simulink model "testSysObj"  (R2013b)
settings: Solver=FixedStepDiscrete  StartTime=0.0  StopTime=Inf  FixedStep=Ts  RelTol=1e-3
PreLoadFcn:
  | s1 = w32serial('COM8');
  | s2 = w32serial('COM40');
  | Ts = 1;
InitFcn:
  | if isequal(s1.CurrentState,'Opened')
  |     fclose(s1);
  | end
  | if isequal(s2.CurrentState,'Opened')
  |     fclose(s2);
  | end
  | 
  | fopen(s1);
  | fopen(s2);
StopFcn:
  | if isequal(s1.CurrentState,'Opened')
  |     fclose(s1);
  | end
  | if isequal(s2.CurrentState,'Opened')
  |     fclose(s2);
  | end
libraries: simulink x2, aerolibanimutils x1
settings Model: Creator=scastro  LastModifiedBy=scastro

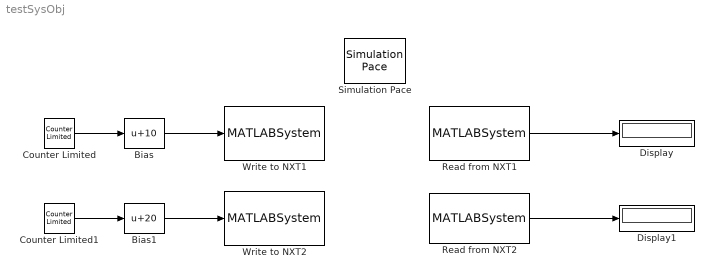
== system testSysObj ==
  Bias : Bias  Bias=10
  Bias1 : Bias  Bias=20
  Counter Limited : simulink/Sources/Counter Limited  uplimit=7  tsamp=Ts
  Counter Limited1 : simulink/Sources/Counter Limited  uplimit=7  tsamp=Ts
  Display : Display
  Display1 : Display
  Read from NXT1 : MATLABSystem  System=w32read  SimulateUsing=Interpreted execution  COMObj=s1  DataType=uint8  DataSize=1  DataLength=1  Mailbox=2
      mask Type: w32read
      mask Display:
      | disp('w32read');
      | port_label('output',1,'msg');
  Read from NXT2 : MATLABSystem  System=w32read  SimulateUsing=Interpreted execution  COMObj=s2  DataType=uint8  DataSize=1  DataLength=1  Mailbox=4
      mask Type: w32read
      mask Display:
      | disp('w32read');
      | port_label('output',1,'msg');
  Simulation Pace : aerolibanimutils/Simulation Pace  SimulationPace=1  SleepMode=MATLAB Thread  OutputPaceError=off  SampleTime=-1
      settings: AttributesFormatString=%<SimulationPace> sec/sec
  Write to NXT1 : MATLABSystem  System=w32write  SimulateUsing=Interpreted execution  COMObj=s1  DataType=uint8  DataSize=1  DataLength=1  Mailbox=1
      mask Type: w32write
      mask Display:
      | disp('w32write');
      | port_label('input',1,'data');
  Write to NXT2 : MATLABSystem  System=w32write  SimulateUsing=Interpreted execution  COMObj=s2  DataType=uint8  DataSize=1  DataLength=1  Mailbox=3
      mask Type: w32write
      mask Display:
      | disp('w32write');
      | port_label('input',1,'data');
  wires:
  Counter Limited/1 -> Bias/1
  Bias1/1 -> Write to NXT2/1
  Counter Limited1/1 -> Bias1/1
  Bias/1 -> Write to NXT1/1
  Read from NXT1/1 -> Display/1
  Read from NXT2/1 -> Display1/1
